simulink model "state_press_zuiyou_15"  (R2018b)
settings: Solver=VariableStepAuto  StartTime=0.0  StopTime=40  RelTol=1e-3  EnableMultiTasking=on
settings Model: Creator=B303  LastModifiedBy=erange
settings DataIOCC: LimitDataPoints=on
settings OptimizationCC: LifeSpan=inf
settings DebuggingCC: AllowSymbolicDim=off  SFUnexpectedBacktrackingDiag=warning  SFNoUnconditionalDefaultTransitionDiag=warning  SFExecutionAtInitializationDiag=none
settings ModelReferenceCC: PropagateSignalLabelsOutOfModel=off
settings SFSimCC: SimUseLocalCustomCode=off
settings RTWCC: RTWUseLocalCustomCode=off
settings CodeAppCC: StateflowObjectComments=on
settings GRTTargetCC: TargetLangStandard=C89/C90 (ANSI)
settings ConfigComp: CovMetricSettings=dw  CovHtmlReporting=on  CovSaveCumulativeToWorkspaceVar=on  CovSaveSingleToWorkspaceVar=on  CovExternalEMLEnable=off

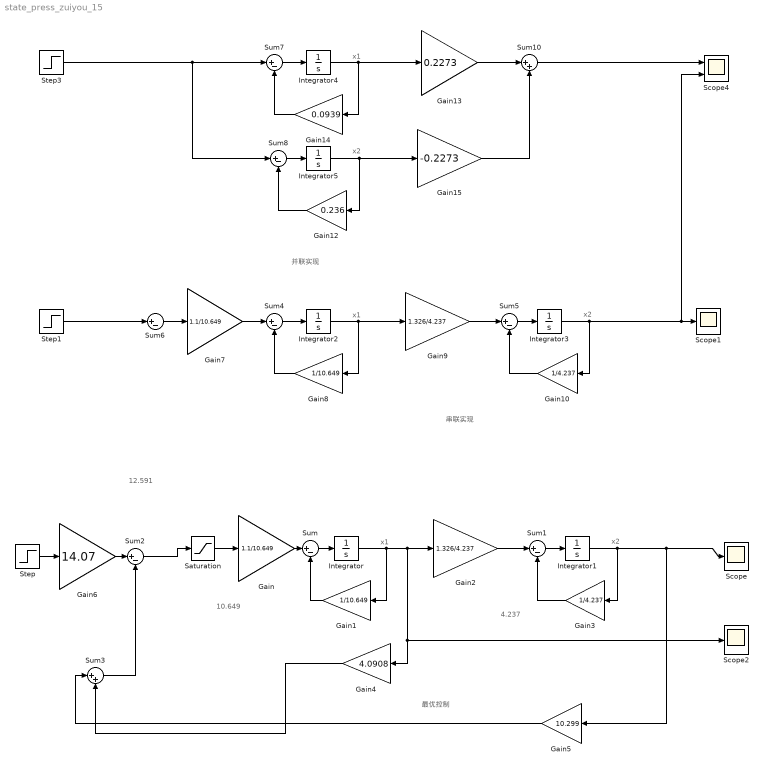
== system state_press_zuiyou_15 ==
  note: 最优控制
  note: 4.237
  note: 10.649
  note: 12.591
  note: 并联实现
  note: 串联实现
  note: x1
  note: x2
  note: x1
  note: x2
  note: x2
  note: x1
  Gain : Gain  Gain=1.1/10.649
  Gain1 : Gain  Gain=1/10.649
  Gain10 : Gain  Gain=1/4.237
  Gain12 : Gain  Gain=0.236
  Gain13 : Gain  Gain=0.2273
  Gain14 : Gain  Gain=0.0939
  Gain15 : Gain  Gain=-0.2273
  Gain2 : Gain  Gain=1.326/4.237
  Gain3 : Gain  Gain=1/4.237
  Gain4 : Gain  Gain=4.0908
  Gain5 : Gain  Gain=10.299
  Gain6 : Gain  Gain=14.07
  Gain7 : Gain  Gain=1.1/10.649
  Gain8 : Gain  Gain=1/10.649
  Gain9 : Gain  Gain=1.326/4.237
  Integrator{,1..5} (6 alike) : Integrator
  Saturation : Saturate  UpperLimit=5  LowerLimit=0
  Scope : Scope
  Scope1 : Scope
  Scope2 : Scope
  Scope4 : Scope  NumInputPorts=2
  Step : Step  Time=0  SampleTime=0
  Step1 : Step  Time=0  SampleTime=0
  Step3 : Step  Time=0  SampleTime=0
  Sum{,1..2,4..8} (8 alike) : Sum  Inputs=|+-
  Sum10 : Sum  Inputs=|++
  Sum3 : Sum  Inputs=|++
  wires:
  Sum/1 -> Integrator/1
  Gain/1 -> Sum/1
  Integrator/1 -> Gain1/1, Scope2/1, Gain4/1, Gain2/1
  Gain2/1 -> Sum1/1
  Sum1/1 -> Integrator1/1
  Sum3/1 -> Sum2/2
  Gain5/1 -> Sum3/1
  Gain4/1 -> Sum3/2
  Step/1 -> Gain6/1
  Gain6/1 -> Sum2/1
  Step1/1 -> Sum6/1
  Sum5/1 -> Integrator3/1
  Sum6/1 -> Gain7/1
  Integrator2/1 -> Gain8/1, Gain9/1
  Sum4/1 -> Integrator2/1
  Integrator3/1 -> Gain10/1, Scope4/2, Scope1/1
  Gain10/1 -> Sum5/2
  Gain9/1 -> Sum5/1
  Gain7/1 -> Sum4/1
  Gain8/1 -> Sum4/2
  Gain1/1 -> Sum/2
  Gain3/1 -> Sum1/2
  Integrator1/1 -> Gain3/1, Gain5/1, Scope/1
  Gain14/1 -> Sum7/2
  Gain12/1 -> Sum8/2
  Sum7/1 -> Integrator4/1
  Integrator5/1 -> Gain15/1, Gain12/1
  Sum8/1 -> Integrator5/1
  Integrator4/1 -> Gain13/1, Gain14/1
  Gain13/1 -> Sum10/1
  Gain15/1 -> Sum10/2
  Step3/1 -> Sum8/1, Sum7/1
  Sum10/1 -> Scope4/1
  Sum2/1 -> Saturation/1
  Saturation/1 -> Gain/1
